simulink model "POSINP"  (R2022b)
settings: configuration reference "SharedConfig" (kept outside this file)
values from neighbouring files (symbols this model uses):
  DT_POSINP_C = 0.0001    [POSINP.sldd]
  EncoderCtPerRev_C = 1000.0    [POSINP.sldd]
  EncoderOfs_C = 0.0    [POSINP.sldd]
  MotPolePairs_C = 4.0    [POSINP.sldd]
  MotPosnEstimrGainI_C = 0.0    [POSINP.sldd]
  MotPosnEstimrGainP_C = 0.0    [POSINP.sldd]
  MotPosnEstimrIntglEna_C = 0.0    [POSINP.sldd]
  MotPosnMagDialEna_C = 1.0    [POSINP.sldd]
  MotPosnMagDialVal_C = 0.0    [POSINP.sldd]
  MotPosnOfs_C = 0.0    [POSINP.sldd]
  MotPosnSenMeth_C = 1.0    [POSINP.sldd]
  MotSpdDialEna_C = 1.0    [POSINP.sldd]
  MotSpdDialVal_C = 0.0    [POSINP.sldd]
  MotSpdFilTiCon_C = 0.001    [POSINP.sldd]
  MotSpdMagDialEna_C = 1.0    [POSINP.sldd]
  MotSpdMagDialVal_C = 0.0    [POSINP.sldd]
undefined symbols (not defined in the file or in its folder): DiscIntNeverNeededParam, DRIVEMODE, slcm
libraries: simulink x2, BlockLibrary x1
Description:
  | Determines the rotor position and speed.
settings Model: DataDictionary=POSINP.sldd  Creator=Kevin  LastModifiedBy=Max Kolesnikov
settings ConfigSetRef: SourceName=SharedConfig

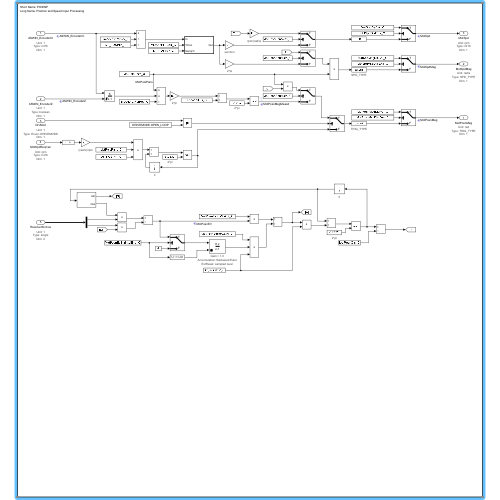
[thumbnail: Simulink's stored preview of the top-level diagram]
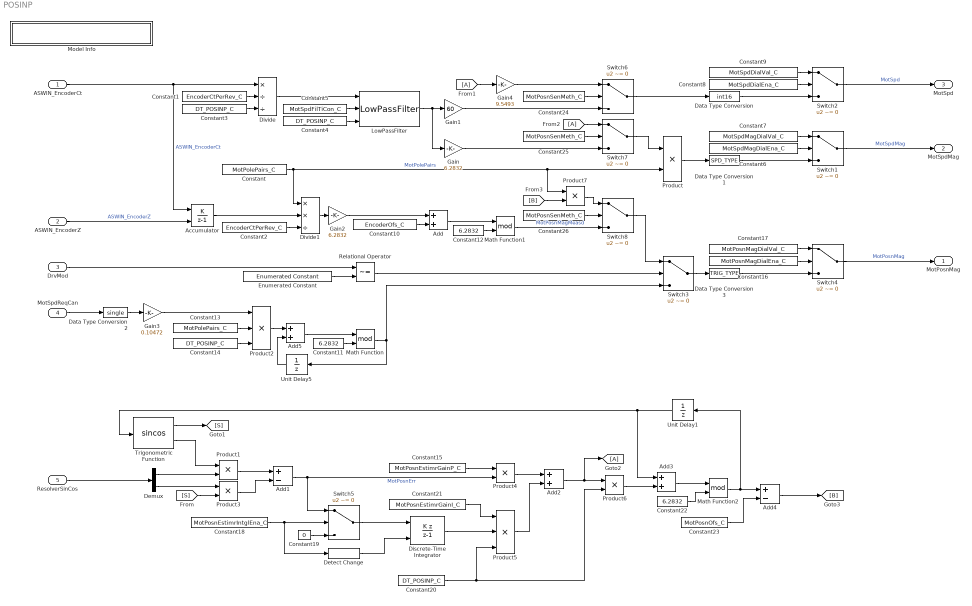
== system POSINP ==
  ASWIN_EncoderCt : Inport  OutDataTypeStr=int16  Unit=1  PortDimensions=1
      settings: AttributesFormatString=|
      | Unit: %<Unit>
      | Type: %<OutDataTypeStr>
      | Dim: %<PortDimensions>
  ASWIN_EncoderZ : Inport  Port=2  OutDataTypeStr=boolean  Unit=1  PortDimensions=1
      settings: AttributesFormatString=|
      | Unit: %<Unit>
      | Type: %<OutDataTypeStr>
      | Dim: %<PortDimensions>
  DrvMod : Inport  Port=3  OutDataTypeStr=Enum: DRIVEMODE  Unit=1  PortDimensions=1
      settings: AttributesFormatString=|
      | Unit: %<Unit>
      | Type: %<OutDataTypeStr>
      | Dim: %<PortDimensions>
  MotSpdReqCan : Inport  Port=4  OutDataTypeStr=int16  Unit=rpm  PortDimensions=1
      settings: AttributesFormatString=|
      | Unit: %<Unit>
      | Type: %<OutDataTypeStr>
      | Dim: %<PortDimensions>
  ResolverSinCos : Inport  Port=5  OutDataTypeStr=single  Unit=1  PortDimensions=2
      settings: AttributesFormatString=|
      | Unit: %<Unit>
      | Type: %<OutDataTypeStr>
      | Dim: %<PortDimensions>
  Accumulator : DiscreteIntegrator  IntegratorMethod=Accumulation: Forward Euler  ExternalReset=rising  SampleTime=-1  OutDataTypeStr=int32  ICPrevOutput=DiscIntNeverNeededParam  ICPrevScaledInput=DiscIntNeverNeededParam
  Add : Sum
  Add1 : Sum  Inputs=+-
  Add2 : Sum
  Add3 : Sum
  Add4 : Sum  Inputs=+-
  Add5 : Sum  OutDataTypeStr=Inherit: Same as first input
  Constant : Constant  Value=MotPolePairs_C
  Constant1 : Constant  Value=EncoderCtPerRev_C
  Constant10 : Constant  Value=EncoderOfs_C
  Constant11 : Constant  Description=2*pi  Value=6.2832  OutDataTypeStr=single
      settings: AttributesFormatString=%<Description>
  Constant12 : Constant  Description=2*pi  Value=6.2832  OutDataTypeStr=single
      settings: AttributesFormatString=%<Description>
  Constant13 : Constant  Value=MotPolePairs_C
  Constant14 : Constant  Value=DT_POSINP_C  VectorParams1D=off
  Constant15 : Constant  Value=MotPosnEstimrGainP_C
  Constant16 : Constant  Value=MotPosnMagDialEna_C
  Constant17 : Constant  Value=MotPosnMagDialVal_C
  Constant18 : Constant  Value=MotPosnEstimrIntglEna_C
  Constant19 : Constant  Value=0  OutDataTypeStr=single
      settings: AttributesFormatString=%<Description>
  Constant2 : Constant  Value=EncoderCtPerRev_C
  Constant20 : Constant  Value=DT_POSINP_C  VectorParams1D=off
  Constant21 : Constant  Value=MotPosnEstimrGainI_C
  Constant22 : Constant  Description=2*pi  Value=6.2832  OutDataTypeStr=single
      settings: AttributesFormatString=%<Description>
  Constant23 : Constant  Value=MotPosnOfs_C  VectorParams1D=off
  Constant24 : Constant  Value=MotPosnSenMeth_C
  Constant25 : Constant  Value=MotPosnSenMeth_C
  Constant26 : Constant  Value=MotPosnSenMeth_C
  Constant3 : Constant  Value=DT_POSINP_C  VectorParams1D=off
  Constant4 : Constant  Value=DT_POSINP_C
  Constant5 : Constant  Value=MotSpdFilTiCon_C
  Constant6 : Constant  Value=MotSpdMagDialEna_C
  Constant7 : Constant  Value=MotSpdMagDialVal_C
  Constant8 : Constant  Value=MotSpdDialEna_C
  Constant9 : Constant  Value=MotSpdDialVal_C
  Data Type Conversion : DataTypeConversion  OutDataTypeStr=int16  SaturateOnIntegerOverflow=off  RndMeth=Floor
  Data Type Conversion1 : DataTypeConversion  OutDataTypeStr=SPD_TYPE  SaturateOnIntegerOverflow=off  RndMeth=Floor
      settings: AttributesFormatString=%<OutDataTypeStr>
  Data Type Conversion2 : DataTypeConversion  OutDataTypeStr=single  SaturateOnIntegerOverflow=off  RndMeth=Floor
  Data Type Conversion3 : DataTypeConversion  OutDataTypeStr=TRIG_TYPE  SaturateOnIntegerOverflow=off  RndMeth=Floor
      settings: AttributesFormatString=%<OutDataTypeStr>
  Demux : Demux  Outputs=2
  Detect Change : simulink/Logic and Bit Operations/Detect Change  vinit=0  OutDataTypeStr=boolean
  Discrete-Time Integrator : DiscreteIntegrator  IntegratorMethod=Accumulation: Backward Euler  ExternalReset=sampled level  SampleTime=-1  OutDataTypeStr=single  ICPrevOutput=DiscIntNeverNeededParam  ICPrevScaledInput=DiscIntNeverNeededParam
      settings: AttributesFormatString=|
      | Gain = %<gainval>
      | %<IntegratorMethod>
      | ExtReset: %<ExternalReset>
  Divide : Product  Inputs=*//  OutDataTypeStr=single
  Divide1 : Product  Inputs=**/  OutDataTypeStr=single
  Enumerated Constant : simulink/Sources/Enumerated Constant  OutDataTypeStr=Enum: DRIVEMODE  Value=DRIVEMODE.OPEN_LOOP  SampleTime=inf
  From1 : From
  From2 : From
  Gain : Gain  Description=2*pi  Gain=6.2832  OutDataTypeStr=Inherit: Same as input  ParamDataTypeStr=Inherit: Same as input
      settings: AttributesFormatString=%<Description>
  Gain1 : Gain  Description=sec/min  Gain=60  OutDataTypeStr=Inherit: Same as input  ParamDataTypeStr=Inherit: Same as input
      settings: AttributesFormatString=%<Description>
  Gain2 : Gain  Description=2*pi  Gain=6.2832  OutDataTypeStr=Inherit: Same as input  ParamDataTypeStr=Inherit: Same as input
      settings: AttributesFormatString=%<Description>
  Gain3 : Gain  Description=(rad/s)/rpm  Gain=0.10472  OutDataTypeStr=Inherit: Same as input  ParamDataTypeStr=Inherit: Same as input
      settings: AttributesFormatString=%<Description>
  Gain4 : Gain  Description=rpm/(rad/s)  Gain=9.5493  OutDataTypeStr=Inherit: Same as input  ParamDataTypeStr=Inherit: Same as input
      settings: AttributesFormatString=%<Description>
  Goto2 : Goto
  LowPassFilter : BlockLibrary/LowPassFilter  SystemSampleTime=-1  VariantActivationTime=update diagram  Latency=0  AutoFrameSizeCalculation=off
  Math Function : Math  Operator=mod
  Math Function1 : Math  Operator=mod
  Math Function2 : Math  Operator=mod
  Model Info : Subsystem  LoadFcn=slcm LoadBlock;  InitFcn=slcm('UpdateAllCMBlocksInThisModelInit')  mask(CMBlock){Frame=off, DisplayStringWithTags=|, MaskDisplayString=Short Name: POSINP\nLong Name: Position and Speed Input Processing, HorizontalTextAlignment=Left, LeftAlignmentValue=0.02}
      mask DisplayStringWithTags=|
      | Short Name: %<ModelName>
      | Long Name: Position and Speed Input Processing
      mask prompts: Frame "Simulink:masks:Frame_MP"; DisplayStringWithTags "Simulink:masks:DisplayStringWithTags_MP"; MaskDisplayString "Simulink:masks:MaskDisplayString_MP"; HorizontalTextAlignment "Simulink:masks:HorizontalTextAlignment_MP"; LeftAlignmentValue "Simulink:masks:LeftAlignmentValue_MP"
      mask help: Simulink:masks:CMBlock_MD
      settings: CopyFcn=slcm CopyBlock;  DeleteFcn=slcm Cancel;  PostSaveFcn=slcm('UpdateAllCMBlocksInThisModel')  NameChangeFcn=slcm Rename;  OpenFcn=slcm
      mask Display: text(slResolve(LeftAlignmentValue, gcbh), 0.5, MaskDisplayString, 'HorizontalAlignment', HorizontalTextAlignment)
  Product{,1,3..4,6..7} (6 alike) : Product
  Product2 : Product  Inputs=***  OutDataTypeStr=single
  Product5 : Product  Inputs=***  OutDataTypeStr=single
  Relational Operator : RelationalOperator  Operator=~=  OutDataTypeStr=boolean  RndMeth=Simplest  InputSameDT=off
  Switch{1..8} (8 alike) : Switch  Criteria=u2 ~= 0  SaturateOnIntegerOverflow=off  InputSameDT=off
  Trigonometric Function : Trigonometry  Operator=sincos  OutputSignalType=real
  Unit Delay1 : UnitDelay  SampleTime=-1  HasFrameUpgradeWarning=on
      settings: AttributesFormatString=%<InitialCondition>
  Unit Delay5 : UnitDelay  SampleTime=-1  HasFrameUpgradeWarning=on
      settings: AttributesFormatString=%<InitialCondition>
  MotPosnMag : Outport  OutDataTypeStr=TRIG_TYPE  Unit=rad  PortDimensions=1
      settings: AttributesFormatString=|
      | Unit: %<Unit>
      | Type: %<OutDataTypeStr>
      | Dim: %<PortDimensions>
  MotSpdMag : Outport  Port=2  OutDataTypeStr=SPD_TYPE  Unit=rad/s  PortDimensions=1
      settings: AttributesFormatString=|
      | Unit: %<Unit>
      | Type: %<OutDataTypeStr>
      | Dim: %<PortDimensions>
  MotSpd : Outport  Port=3  OutDataTypeStr=int16  Unit=rpm  PortDimensions=1
      settings: AttributesFormatString=|
      | Unit: %<Unit>
      | Type: %<OutDataTypeStr>
      | Dim: %<PortDimensions>
  wires:
  Switch4/1 -> MotPosnMag/1  "MotPosnMag"
  ASWIN_EncoderZ/1 -> Accumulator/2  "ASWIN_EncoderZ"
  Constant/1 -> Divide1/1, Product7/1, Product/2  "MotPolePairs"
  ASWIN_EncoderCt/1 -> Divide/1, Accumulator/1  "ASWIN_EncoderCt"
  Constant1/1 -> Divide/2
  Constant3/1 -> Divide/3
  Divide/1 -> LowPassFilter/1
  Constant4/1 -> LowPassFilter/3
  Constant5/1 -> LowPassFilter/2
  LowPassFilter/1 -> Gain/1, Gain1/1
  Constant2/1 -> Divide1/3
  Accumulator/1 -> Divide1/2
  Divide1/1 -> Gain2/1
  Gain2/1 -> Add/1
  Constant16/1 -> Switch4/2
  Constant17/1 -> Switch4/1
  Constant7/1 -> Switch1/1
  Constant6/1 -> Switch1/2
  Constant8/1 -> Switch2/2
  Constant9/1 -> Switch2/1
  Gain1/1 -> Switch6/3
  Switch1/1 -> MotSpdMag/1  "MotSpdMag"
  Switch2/1 -> MotSpd/1  "MotSpd"
  Constant10/1 -> Add/2
  Data Type Conversion/1 -> Switch2/3
  Data Type Conversion1/1 -> Switch1/3
  DrvMod/1 -> Relational Operator/1
  Relational Operator/1 -> Switch3/2
  Switch3/1 -> Data Type Conversion3/1
  Add/1 -> Math Function1/1
  Math Function1/1 -> Switch8/3  "MotPosnMagMeasd"
  MotSpdReqCan/1 -> Data Type Conversion2/1
  Unit Delay5/1 -> Add5/2
  Math Function/1 -> Switch3/3, Unit Delay5/1
  Product2/1 -> Add5/1
  Constant14/1 -> Product2/3
  Gain3/1 -> Product2/1
  Data Type Conversion2/1 -> Gain3/1
  Constant11/1 -> Math Function/2
  Add5/1 -> Math Function/1
  Constant12/1 -> Math Function1/2
  ResolverSinCos/1 -> Demux/1
  Demux/1 -> Product1/2
  Demux/2 -> Product3/1
  Trigonometric Function/2 -> Product1/1
  Trigonometric Function/1 -> [S]
  [S] -> Product3/2
  Constant13/1 -> Product2/2
  Enumerated Constant/1 -> Relational Operator/2
  Product1/1 -> Add1/1
  Product3/1 -> Add1/2
  Unit Delay1/1 -> Add3/1, Trigonometric Function/1
  Add1/1 -> Switch5/1, Product4/2  "MotPosnErr"
  Constant15/1 -> Product4/1
  Product4/1 -> Add2/1
  Constant18/1 -> Detect Change/1, Switch5/2
  Constant19/1 -> Switch5/3
  Switch5/1 -> Discrete-Time Integrator/1
  Detect Change/1 -> Discrete-Time Integrator/2
  Constant20/1 -> Product6/2, Product5/3
  Discrete-Time Integrator/1 -> Product5/2
  Constant21/1 -> Product5/1
  Product5/1 -> Add2/2
  Add2/1 -> Product6/1, Goto2/1
  Product6/1 -> Add3/2
  Constant22/1 -> Math Function2/2
  Add3/1 -> Math Function2/1
  Math Function2/1 -> Unit Delay1/1, Add4/1
  Constant23/1 -> Add4/2
  Switch6/1 -> Data Type Conversion/1
  Constant24/1 -> Switch6/2
  Constant25/1 -> Switch7/2
  Product/1 -> Data Type Conversion1/1
  Constant26/1 -> Switch8/2
  Switch8/1 -> Switch3/1
  From1/1 -> Gain4/1
  Gain4/1 -> Switch6/1
  Switch7/1 -> Product/1
  Gain/1 -> Switch7/3
  From2/1 -> Switch7/1
  Product7/1 -> Switch8/1
  Add4/1 -> [B]
  [B] -> Product7/2
  Data Type Conversion3/1 -> Switch4/3

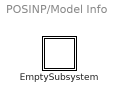
== system POSINP/Model Info ==
  EmptySubsystem : Subsystem

== system POSINP/Model Info/EmptySubsystem ==
